simulink model "MPSLab4"  (R2014b)
settings: Solver=ode45  StartTime=0.0  StopTime=10.0  RelTol=1e-3
settings Model: Creator=kiril_000  LastModifiedBy=kiril_000

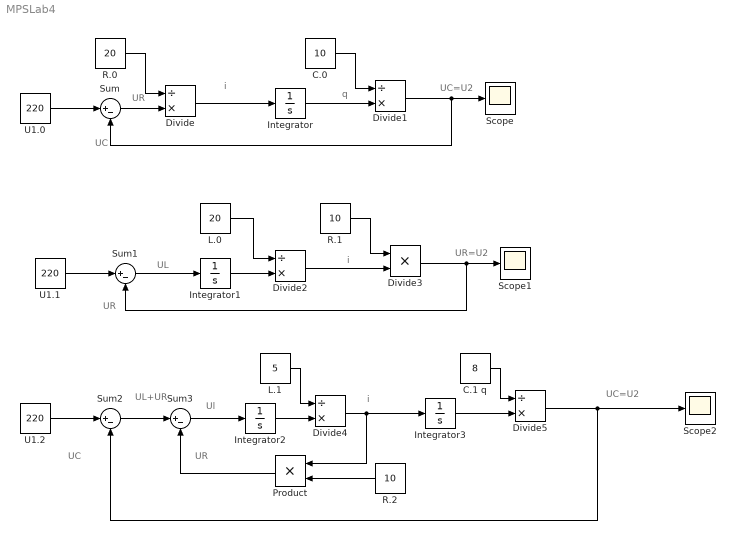
== system MPSLab4 ==
  note: UC
  note: UC=U2
  note: UL+UR
  note: UR
  note: Ul
  note: i
  note: UR
  note: UC
  note: UC=U2
  note: q
  note: UR
  note: i
  note: UR=U2
  note: UL
  note: i
  C.0 : Constant  Value=10
  C.1 q : Constant  Value=8
  Divide{,1..2,4..5} (5 alike) : Product  Inputs=/*
  Divide3 : Product  Inputs=**
  Integrator{,1..3} (4 alike) : Integrator
  L.0 : Constant  Value=20
  L.1 : Constant  Value=5
  Product : Product
  R.0 : Constant  Value=20
  R.1 : Constant  Value=10
  R.2 : Constant  Value=10
  Scope : Scope
  Scope1 : Scope
  Scope2 : Scope
      settings: SaveName=ScopeData2
  Sum{,1..3} (4 alike) : Sum  Inputs=|+-
  U1.0 : Constant  Value=220
  U1.1 : Constant  Value=220
  U1.2 : Constant  Value=220
  wires:
  U1.0/1 -> Sum/1
  R.0/1 -> Divide/1
  Sum/1 -> Divide/2
  Divide/1 -> Integrator/1
  Integrator/1 -> Divide1/2
  C.0/1 -> Divide1/1
  Divide1/1 -> Sum/2, Scope/1
  U1.1/1 -> Sum1/1
  L.0/1 -> Divide2/1
  R.1/1 -> Divide3/1
  Divide3/1 -> Scope1/1, Sum1/2
  Sum1/1 -> Integrator1/1
  Integrator1/1 -> Divide2/2
  Divide2/1 -> Divide3/2
  Divide4/1 -> Product/1, Integrator3/1
  Integrator3/1 -> Divide5/2
  Integrator2/1 -> Divide4/2
  L.1/1 -> Divide4/1
  C.1 q/1 -> Divide5/1
  R.2/1 -> Product/2
  Sum3/1 -> Integrator2/1
  Product/1 -> Sum3/2
  Sum2/1 -> Sum3/1
  U1.2/1 -> Sum2/1
  Divide5/1 -> Sum2/2, Scope2/1
